simulink model "controller13_AIS"  (R2020b)
settings: Solver=FixedStepDiscrete  StartTime=0.0  StopTime=inf  RelTol=1e-3
values from neighbouring files (symbols this model uses):
  ctr = make_controller()    [setup_controller_with_functions.m]
  mdl = make_model(flight_time)    [setup_controller_with_functions.m]
  ukf_P0_flat = UKF.flatten_matrix(ukf_sys.P0)    [controller_setup_ukf.m]
  ukf_prediction_time = 0.015    [controller_setup_ukf.m]
  ukf_s0 = ukf_sys.s0    [controller_setup_ukf.m]
  ukf_sys = UKF.initialize_ukf_sys(rbt, mdl, ukf_params)    [controller_setup_ukf.m]
  ukf_use_prediction = 1    [controller_setup_ukf.m]
undefined symbols (not defined in the file or in its folder): ctr1, ctr2, DiscIntNeverNeededParam, flt, IO397, rbt1, rbt2, rsim1, rsim2, som, traj2
libraries: simulink x63, slrealtimeloglib x21, slrealtimetgmanagement x8, slrealtimeseriallib x5, speedgoatlib_fpga_analog_io x4, slrealtimeutilitieslib x3, dspfdesign x2, speedgoatlib_fpga x2, slrealtimeiplib x2, speedgoatlib_fpga_dio x1
(part 1 of 5)
settings Model: SimulationMode=external  Creator=SMRL  LastModifiedBy=SMRL
settings SolverCC: ConcurrentTasks=on  PositivePriorityOrder=on  AutoInsertRateTranBlk=on
settings DataIOCC: DSMLogging=off
settings OptimizationCC: BlockReduction=off  OptimizeBlockIOStorage=off
settings DebuggingCC: TasksWithSamePriorityMsg=none
settings HardwareCC: ProdBitPerLong=64  ProdLongLongMode=on  ProdHWDeviceType=Intel->x86-64 (Linux 64)
settings RTWCC: Description=Simulink Real-Time  SystemTargetFile=slrealtime.tlc  TemplateMakefile=slrealtime_default_tmf  Toolchain=Simulink Real-Time Toolchain  BuildConfiguration=Faster Runs  CodeExecutionProfiling=on  CodeProfilingInstrumentation=coarse  TargetLang=C++

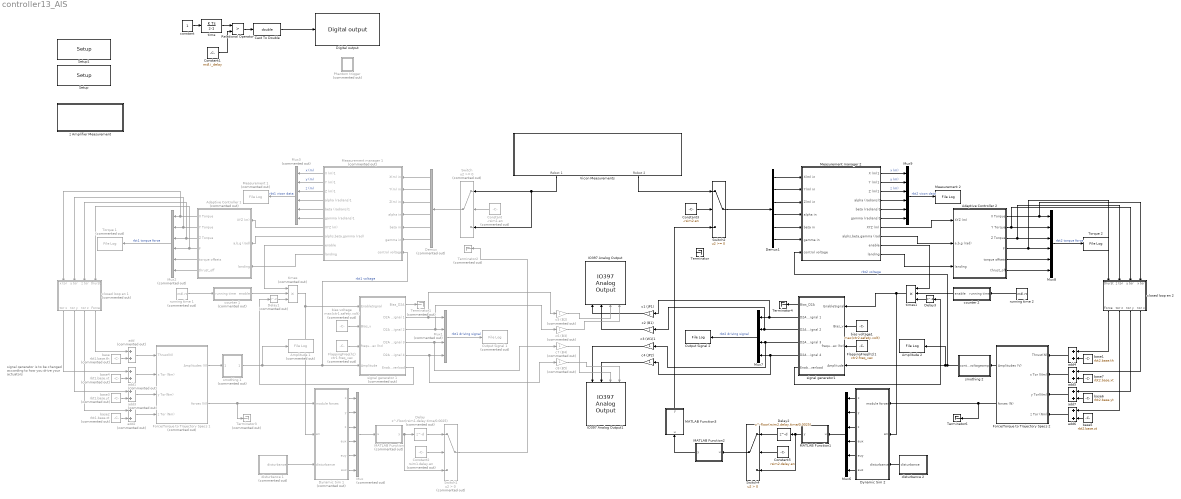
== system controller13_AIS ==
  note: signal generator is to be changed
      | according to how you drive your
      | actuators
  Adaptive Controller 1 : Subsystem  Commented=on
  Adaptive Controller 2 : Subsystem
  Amplitude 1 : slrealtimeloglib/File Log  Commented=on  decimation=1
      settings: SourceProductBaseCode=XP
  Amplitude 2 : slrealtimeloglib/File Log  decimation=1
      settings: SourceProductBaseCode=XP
  Cast To Double : DataTypeConversion  OutDataTypeStr=double
  Constant : Constant  Commented=on  Value=-rsim1.en
  Constant1 : Constant  Value=mdl.i_delay
  Constant2 : Constant  Commented=on  Value=rsim1.delay.en
  Constant3 : Constant  Value=-rsim2.en
  Constant5 : Constant  Value=rsim2.delay.en
  Delay : Delay  Commented=on  DelayLength=floor(rsim1.delay.time/0.0025)
  Delay1 : Delay  Commented=on  InitialCondition=1
  Delay2 : Delay  DelayLength=floor(rsim2.delay.time/0.0025)
  Delay3 : Delay  InitialCondition=1
  Demux : Demux  Commented=on  Outputs=6
  Demux1 : Demux  Outputs=6
  Digital output : speedgoatlib_fpga_dio/Digital output  id=2  chan=[7]  init=[0]  reset=[0]  vectorizeInput=off  ts=mdl.T  pciSlot=[11,0]  board=IO397-50k
      settings: SourceProductName=Simulink Real-Time: Speedgoat I/O Driver Library
  Dynamic Sim 1 : Subsystem  Commented=on  TreatAsAtomicUnit=on  SystemSampleTime=rsim1.mdl.T
  Dynamic Sim 2 : Subsystem  TreatAsAtomicUnit=on  SystemSampleTime=rsim2.mdl.T
  FlappingFreq(hz) : Constant  Commented=on  Value=ctr1.freq_vec  SampleTime=-1
  FlappingFreq(hz)1 : Constant  Value=ctr2.freq_vec  SampleTime=-1
  Force/Torque to Trajectory Specs 1 : Subsystem  Commented=on
  Force/Torque to Trajectory Specs 2 : Subsystem
  IO397 Analog Output : speedgoatlib_fpga_analog_io/IO397 Analog Output  id=1  chan=1:4  initVal=0  resetVal=0  ts=-1  pciSlot=[6,0]  board=IO397-50k  span=+10.8 V
      settings: SourceProductName=Simulink Real-Time: Speedgoat Library
  IO397 Analog Output1 : speedgoatlib_fpga_analog_io/IO397 Analog Output  id=2  chan=1:4  initVal=0  resetVal=0  ts=-1  pciSlot=[11,0]  board=IO397-50k  span=+10.8 V
      settings: SourceProductName=Simulink Real-Time: Speedgoat Library
  MATLAB Function : MATLAB Function  Commented=on  TreatAsAtomicUnit=on  SystemSampleTime=0.0025
  MATLAB Function1 : MATLAB Function  TreatAsAtomicUnit=on  SystemSampleTime=0.002
  MATLAB Function2 : MATLAB Function  TreatAsAtomicUnit=on  SystemSampleTime=1/500
  MATLAB Function3 : MATLAB Function  TreatAsAtomicUnit=on  SystemSampleTime=mdl.T
  Measurement 1 : slrealtimeloglib/File Log  Commented=on  decimation=1
      settings: SourceProductBaseCode=XP
  Measurement 2 : slrealtimeloglib/File Log  decimation=1
      settings: SourceProductBaseCode=XP
  Measurement manager 1 : Subsystem  Commented=on
  Measurement manager 2 : Subsystem  SystemSampleTime=mdl.T
  Mux : Mux  Commented=on  Inputs=6
  Mux1 : Mux  Commented=on
  Mux2 : Mux  Commented=on  Inputs=6
  Mux3 : Mux  Commented=on  Inputs=6
  Mux6 : Mux  Inputs=6
  Mux7 : Mux
  Mux8 : Mux  Inputs=6
  Mux9 : Mux  Inputs=6
  Output Signal 1 : slrealtimeloglib/File Log  Commented=on  decimation=1
      settings: SourceProductBaseCode=XP
  Output Signal 2 : slrealtimeloglib/File Log  decimation=1
      settings: SourceProductBaseCode=XP
  Phantom trigger : Subsystem  Commented=on
  Relational Operator : RelationalOperator  Operator=>  OutDataTypeStr=boolean  RndMeth=Simplest
  Setup : speedgoatlib_fpga/Setup/Setup  board=IO397-50k  id=2  device_id=2  frontIO=None  rearIO=None  bitstreamFile=speedgoat_IO397_50k_all_io_2.mat  rev=2.1  timestamp_string=06/12/19 11:07:30  fpgaFreq=75 MHz  fpgaTick=13.33 ns  ProgSpiFlash=off  ProgBPIFlash=off  pciSlot=[11,0]  PullRPort0=pull-up 3.3V  VioPort0=3.3V  PullRPort1=pull-up 3.3V  VioPort1=3.3V  PullRPort2=pull-up 3.3V  VioPort2=3.3V  PullRPort3=pull-up 3.3V  VioPort3=3.3V  PullRPort4=pull-up 3.3V  VioPort4=3.3V  PullRPort5=pull-up 3.3V  VioPort5=3.3V  PullRPort6=pull-up 3.3V  VioPort6=3.3V  PullRPort15=pull-up 3.3V  PullRPort31=pull-up 3.3V  PullRPort47=pull-up 3.3V  PullRPort63=pull-up 3.3V
      settings: SourceProductName=Simulink Real-Time: Speedgoat Library
  Setup1 : speedgoatlib_fpga/Setup/Setup  board=IO397-50k  id=1  device_id=1  frontIO=None  rearIO=None  bitstreamFile=speedgoat_IO397_50k_all_io_2.mat  rev=2.1  timestamp_string=06/12/19 11:07:30  fpgaFreq=75 MHz  fpgaTick=13.33 ns  ProgSpiFlash=off  ProgBPIFlash=off  pciSlot=[6,0]  PullRPort0=pull-up 3.3V  VioPort0=3.3V  PullRPort1=pull-up 3.3V  VioPort1=3.3V  PullRPort2=pull-up 3.3V  VioPort2=3.3V  PullRPort3=pull-up 3.3V  VioPort3=3.3V  PullRPort4=pull-up 3.3V  VioPort4=3.3V  PullRPort5=pull-up 3.3V  VioPort5=3.3V  PullRPort6=pull-up 3.3V  VioPort6=3.3V  PullRPort15=pull-up 3.3V  PullRPort31=pull-up 3.3V  PullRPort47=pull-up 3.3V  PullRPort63=pull-up 3.3V
      settings: SourceProductName=Simulink Real-Time: Speedgoat Library
  Switch : Switch  Commented=on
  Switch1 : Switch  Commented=on  Criteria=u2 > Threshold
  Switch2 : Switch
  Switch4 : Switch  Criteria=u2 > Threshold
  Terminator : Terminator
  Terminator1 : Terminator  Commented=on
  Terminator2 : Terminator  Commented=on
  Terminator3 : Terminator  Commented=on
  Terminator4 : Terminator
  Terminator6 : Terminator
  Torque 1 : slrealtimeloglib/File Log  Commented=on  decimation=1
      settings: SourceProductBaseCode=XP
  Torque 2 : slrealtimeloglib/File Log  decimation=1
      settings: SourceProductBaseCode=XP
  Vicon Measurements : Subsystem
  add{,1..3} (4 alike) : Sum  Commented=on
  add{4..7} (4 alike) : Sum
  base : Constant  Commented=on  Value=rbt1.base.th
  base1 : Constant  Value=rbt2.base.th
  base2 : Constant  Commented=on  Value=rbt1.base.zt
  base3 : Constant  Commented=on  Value=rbt1.base.yt
  base4 : Constant  Commented=on  Value=rbt1.base.xt
  base5 : Constant  Value=rbt2.base.zt
  base6 : Constant  Value=rbt2.base.yt
  base7 : Constant  Value=rbt2.base.xt
  bias voltage : Constant  Commented=on  Value=max(ctr1.safety.volt)
  bias voltage1 : Constant  Value=max(ctr2.safety.volt)
  c1 (JP1) : Gain
  c2 (B1) : Gain
  c3 (W1)1 : Gain
  c4 (JP2) : Gain
  c5 (B2) : Gain  Commented=on
  c6 (B3) : Gain  Commented=on
  c7 (B4) : Gain  Commented=on
  c8 (B5) : Gain  Commented=on
  closed loop en 1 : Subsystem  Commented=on
  closed loop en 2 : Subsystem
  constant : Constant
  counter 1 : Subsystem  Commented=on
  counter 2 : Subsystem
  disturbance 1 : Subsystem  Commented=on  TreatAsAtomicUnit=on  SystemSampleTime=rsim1.mdl.T
  disturbance 2 : Subsystem  TreatAsAtomicUnit=on  SystemSampleTime=rsim2.mdl.T
  running time 1 : Constant  Commented=on  Value=mdl.rt  SampleTime=-1
  running time 2 : Constant  Value=mdl.rt  SampleTime=-1
  signal generator 1 : Subsystem  Commented=on  TreatAsAtomicUnit=on  SystemSampleTime=mdl.T_high
  signal generator1 : Subsystem  TreatAsAtomicUnit=on  SystemSampleTime=mdl.T_high
  smothing 1 : Subsystem  Commented=on
  smothing 2 : Subsystem
  time : DiscreteIntegrator  gainval=1  SampleTime=-1  UpperSaturationLimit=1  LowerSaturationLimit=0  ICPrevOutput=DiscIntNeverNeededParam  ICPrevScaledInput=DiscIntNeverNeededParam
  times : Product  Commented=on  Inputs=3  RndMeth=Zero
  times1 : Product  Inputs=3  RndMeth=Zero
  z Amplifier Measurement : Subsystem
  wires:
  add3/1 -> Force/Torque to Trajectory Specs 1/3(y Tor(Nm))
  Force/Torque to Trajectory Specs 1/2(forces (N)) -> Dynamic Sim 1/1(module forces), Terminator3/1
  Adaptive Controller 1/3(Z Torque) -> Mux2/3, closed loop en 1/3(z tor)
  Mux3/1 -> Measurement 1/1  "rbt1 vicon data"
  Adaptive Controller 1/2(Y Torque) -> Mux2/2, closed loop en 1/2(y tor)
  Adaptive Controller 1/1(X Torque) -> Mux2/1, closed loop en 1/1(x tor)
  signal generator 1/5(D2A DriveSignal 4) -> c8 (B5)/1, Mux1/4
  Adaptive Controller 1/5(" torque offsets") -> Mux2/5
  Measurement manager 1/5(beta (radians)1) -> Mux3/5
  signal generator 1/4(D2A DriveSignal 3) -> c7 (B4)/1, Mux1/3
  Adaptive Controller 1/4(" F") -> Mux2/4, closed loop en 1/4(thurst)
  Measurement manager 1/6(gamma (radians)1) -> Mux3/6
  add2/1 -> Force/Torque to Trajectory Specs 1/4(z Tor (Nm))
  Measurement manager 1/4(alpha (radians)1) -> Mux3/4
  Adaptive Controller 1/6(thrust_off) -> Mux2/6
  closed loop en 1/1(tor x) -> add1/1
  base3/1 -> add3/2
  base2/1 -> add2/2
  Mux1/1 -> Output Signal 1/1  "rbt1 driving signal"
  closed loop en 1/4(Force) -> add/1
  base/1 -> add/2
  Measurement manager 1/8(alphs,beta,gamma (rad)) -> Adaptive Controller 1/2(a,b,g (rad))
  signal generator 1/2(D2A DriveSignal 1) -> Mux1/1, c5 (B2)/1
  closed loop en 1/2(tor y) -> add3/1
  signal generator 1/3(D2A DriveSignal 2) -> c6 (B3)/1, Mux1/2
  Force/Torque to Trajectory Specs 1/1(Amplitudes (V)) -> smothing 1/1(amp)
  FlappingFreq(hz)/1 -> signal generator 1/3(frequency_vec (hz))
  Measurement manager 1/1(X (m)1) -> Mux3/1  "x (m)"
  Measurement manager 1/7(XYZ (m)) -> Adaptive Controller 1/1(XYZ (m))
  Measurement manager 1/3(Z (m)1) -> Mux3/3  "z (m)"
  base4/1 -> add1/2
  closed loop en 1/3(tor z) -> add2/1
  add1/1 -> Force/Torque to Trajectory Specs 1/2(x Tor (Nm))
  bias voltage/1 -> signal generator 1/2(Bias_v)
  counter 1/1(enable) -> times/2
  add/1 -> Force/Torque to Trajectory Specs 1/1(Thrust(N))
  Measurement manager 1/2(Y (m)1) -> Mux3/2  "y (m)"
  running time 1/1 -> counter 1/1(running time)
  Mux2/1 -> Torque 1/1  "rbt1 torque force"
  signal generator 1/1(Bias_D2A) -> Terminator1/1
  Dynamic Sim 1/3(z) -> Mux/3
  Dynamic Sim 1/2(y) -> Mux/2
  Dynamic Sim 1/1(x) -> Mux/1
  Dynamic Sim 1/4(eux) -> Mux/4
  Dynamic Sim 1/5(euy) -> Mux/5
  Dynamic Sim 1/6(euz) -> Mux/6
  Demux/1 -> Measurement manager 1/1(X(m) in)
  Demux/2 -> Measurement manager 1/2(Y(m) in)
  Demux/3 -> Measurement manager 1/3(Z(m) in)
  Demux/4 -> Measurement manager 1/4(alpha in)
  Demux/5 -> Measurement manager 1/5(beta in)
  Demux/6 -> Measurement manager 1/6(gamma in)
  Constant/1 -> Switch/2
  disturbance 1/1(disturbance) -> Dynamic Sim 1/3(disturbance)
  times/1 -> signal generator 1/1(EnableSignal), Dynamic Sim 1/2(en)
  Switch/1 -> Demux/1
  Switch1/1 -> Terminator2/1
  Cast To Double/1 -> Digital output/1
  constant/1 -> time/1
  time/1 -> Relational Operator/1
  Relational Operator/1 -> Cast To Double/1
  Constant1/1 -> Relational Operator/2
  Measurement manager 1/10(landing) -> Adaptive Controller 1/3(landing)
  signal generator 1/6(Enable overload) -> Delay1/1
  Delay1/1 -> times/3
  smothing 1/1(control voltage) -> signal generator 1/4(Amplitude), Measurement manager 1/7(control voltage), Amplitude 1/1  "rbt1 voltage"
  Measurement manager 1/9(enable) -> times/1
  Mux/1 -> MATLAB Function/1(u)
  Delay/1 -> Switch1/1
  Constant2/1 -> Switch1/2
  MATLAB Function/1(y) -> Switch1/3, Delay/1
  Constant3/1 -> Switch2/2
  MATLAB Function1/1(y) -> Switch4/3, Delay2/1
  Mux6/1 -> MATLAB Function1/1(u)
  smothing 2/1(control voltage) -> signal generator1/4(Amplitude), Amplitude 2/1, Measurement manager 2/7(control voltage)  "rbt2 voltage"
  Measurement manager 2/10(landing) -> Adaptive Controller 2/3(landing)
  Demux1/2 -> Measurement manager 2/2(Y(m) in)
  Measurement manager 2/4(alpha (radians)1) -> Mux9/4
  closed loop en 2/2(tor y) -> add7/1
  Demux1/1 -> Measurement manager 2/1(X(m) in)
  Demux1/5 -> Measurement manager 2/5(beta in)
  Delay3/1 -> times1/3
  Delay2/1 -> Switch4/1
  Measurement manager 2/9(enable) -> times1/1
  Constant5/1 -> Switch4/2
  disturbance 2/1(disturbance) -> Dynamic Sim 2/3(disturbance)
  times1/1 -> signal generator1/1(EnableSignal), Dynamic Sim 2/2(en)
  signal generator1/6(Enable overload) -> Delay3/1
  Mux8/1 -> Torque 2/1  "rbt2 torque force"
  signal generator1/3(D2A DriveSignal 2) -> c2 (B1)/1, Mux7/2
  closed loop en 2/3(tor z) -> add6/1
  Demux1/6 -> Measurement manager 2/6(gamma in)
  Dynamic Sim 2/5(euy) -> Mux6/5
  Measurement manager 2/1(X (m)1) -> Mux9/1  "x (m)"
  add6/1 -> Force/Torque to Trajectory Specs 2/4(z Tor (Nm))
  closed loop en 2/1(tor x) -> add5/1
  Dynamic Sim 2/4(eux) -> Mux6/4
  Adaptive Controller 2/6(thrust_off) -> Mux8/6
  Dynamic Sim 2/2(y) -> Mux6/2
  Dynamic Sim 2/1(x) -> Mux6/1
  counter 2/1(enable) -> times1/2
  signal generator1/4(D2A DriveSignal 3) -> c3 (W1)1/1, Mux7/3
  running time 2/1 -> counter 2/1(running time)
  signal generator1/1(Bias_D2A) -> Terminator4/1
  Measurement manager 2/2(Y (m)1) -> Mux9/2  "y (m)"
  Measurement manager 2/5(beta (radians)1) -> Mux9/5
  closed loop en 2/4(Force) -> add4/1
  add4/1 -> Force/Torque to Trajectory Specs 2/1(Thrust(N))
  bias voltage1/1 -> signal generator1/2(Bias_v)
  Adaptive Controller 2/5(" torque offsets") -> Mux8/5
  Dynamic Sim 2/6(euz) -> Mux6/6
  base6/1 -> add7/2
  base5/1 -> add6/2
  Measurement manager 2/6(gamma (radians)1) -> Mux9/6
  base7/1 -> add5/2
  Measurement manager 2/3(Z (m)1) -> Mux9/3  "z (m)"
  Adaptive Controller 2/4(" F") -> Mux8/4, closed loop en 2/4(thurst)
  Measurement manager 2/7(XYZ (m)) -> Adaptive Controller 2/1(XYZ (m))
  Force/Torque to Trajectory Specs 2/2(forces (N)) -> Dynamic Sim 2/1(module forces), Terminator6/1
  Adaptive Controller 2/1(X Torque) -> closed loop en 2/1(x tor), Mux8/1
  add5/1 -> Force/Torque to Trajectory Specs 2/2(x Tor (Nm))
  add7/1 -> Force/Torque to Trajectory Specs 2/3(y Tor(Nm))
  base1/1 -> add4/2
  Mux7/1 -> Output Signal 2/1  "rbt2 driving signal"
  Dynamic Sim 2/3(z) -> Mux6/3
  Mux9/1 -> Measurement 2/1  "rbt2 vicon data"
  Force/Torque to Trajectory Specs 2/1(Amplitudes (V)) -> smothing 2/1(amp)
  Demux1/3 -> Measurement manager 2/3(Z(m) in)
  Measurement manager 2/8(alphs,beta,gamma (rad)) -> Adaptive Controller 2/2(a,b,g (rad))
  Adaptive Controller 2/2(Y Torque) -> closed loop en 2/2(y tor), Mux8/2
  signal generator1/5(D2A DriveSignal 4) -> Mux7/4, c4 (JP2)/1
  Adaptive Controller 2/3(Z Torque) -> closed loop en 2/3(z tor), Mux8/3
  FlappingFreq(hz)1/1 -> signal generator1/3(frequency_vec (hz))
  Demux1/4 -> Measurement manager 2/4(alpha in)
  Switch2/1 -> Demux1/1
  Switch4/1 -> MATLAB Function2/1(u)
  Vicon Measurements/2(Robot 2) -> Switch2/1
  Vicon Measurements/1(Robot 1) -> Switch/3, Switch/1
  signal generator1/2(D2A DriveSignal 1) -> c1 (JP1)/1, Mux7/1
  c1 (JP1)/1 -> IO397 Analog Output/1
  c2 (B1)/1 -> IO397 Analog Output/2
  c3 (W1)1/1 -> IO397 Analog Output1/1
  c4 (JP2)/1 -> IO397 Analog Output1/2
  c5 (B2)/1 -> IO397 Analog Output/3
  c6 (B3)/1 -> IO397 Analog Output/4
  c7 (B4)/1 -> IO397 Analog Output1/3
  c8 (B5)/1 -> IO397 Analog Output1/4
  MATLAB Function2/1(y) -> MATLAB Function3/1(u)
  MATLAB Function3/1(y) -> Switch2/3

== system controller13_AIS/Adaptive Controller 1 ==
  XYZ (m) : Inport
  a,b,g (rad) : Inport  Port=2
  landing : Inport  Port=3
  Mux : Mux
  Overload Options : slrealtimetgmanagement/Overload Options  startupDur=10  startupDurSrc=Tunable Parameter  maxOverload=10  maxOverloadSrc=Tunable Parameter  TETFlag=on
      settings: SourceProductBaseCode=XP
  Terminator : Terminator
  Terminator1 : Terminator
  Terminator2 : Terminator
  adaptive setpoint rd : MATLAB Function  TreatAsAtomicUnit=on  SystemSampleTime=mdl.T
  adaptive system : Subsystem
  attitude and thrust controller : Subsystem
  observer : Subsystem
  observer_log : slrealtimeloglib/File Log  decimation=1
      settings: SourceProductBaseCode=XP
  observer_mux : Mux  Inputs=5
  rd : slrealtimeloglib/File Log  decimation=1
      settings: SourceProductBaseCode=XP
  rd_mux : Mux  Inputs=2
  saturation : MATLAB Function  TreatAsAtomicUnit=on
  somersault_phase : MATLAB Function  TreatAsAtomicUnit=on
  time : Subsystem
  X Torque : Outport
  Y Torque : Outport  Port=2
  Z Torque : Outport  Port=3
  " F" : Outport  Port=4
  " torque offsets" : Outport  Port=5
  thrust_off : Outport  Port=6
  wires:
  XYZ (m)/1 -> observer/1(xyz)
  observer/1(r) -> adaptive setpoint rd/2(r), attitude and thrust controller/1(r)
  observer/2(r_dot) -> observer_mux/1, adaptive setpoint rd/3(r_d), attitude and thrust controller/2(r_dot)
  observer/3(r_dotdot) -> observer_mux/2, attitude and thrust controller/3(r_dotdot)
  a,b,g (rad)/1 -> attitude and thrust controller/12(euler angle), observer/2(euler)
  observer/4(R) -> observer_mux/3, attitude and thrust controller/4(R)
  saturation/1(X_roll) -> Mux/1, X Torque/1
  saturation/2(Y_pitch) -> Mux/2, Y Torque/1
  saturation/3(Z_yaw) -> Mux/3, Z Torque/1
  saturation/4(Force) -> " F"/1, Mux/4
  attitude and thrust controller/4(F) -> saturation/4(Th)
  attitude and thrust controller/5(att_e) -> adaptive system/1(att_e)
  adaptive system/1(" tor_off") -> " torque offsets"/1
  adaptive system/2(th_off) -> thrust_off/1
  adaptive system/3(int_e) -> attitude and thrust controller/11(int_e)
  adaptive setpoint rd/1(rd) -> rd_mux/1, attitude and thrust controller/6(rd)  "rd"
  adaptive setpoint rd/2(rd_d) -> rd_mux/2, attitude and thrust controller/7(rd_d)
  adaptive setpoint rd/3(rd_dd) -> attitude and thrust controller/8(rd_dd)
  adaptive setpoint rd/4(rd_ddd) -> attitude and thrust controller/9(rd_ddd)
  adaptive setpoint rd/5(rd_dddd) -> attitude and thrust controller/10(rd_dddd)
  time/1(real times) -> somersault_phase/1(time), adaptive setpoint rd/1(time)
  attitude and thrust controller/3(torque_z) -> saturation/3(z_yaw)
  attitude and thrust controller/2(torque_y) -> saturation/2(y_pitch)
  attitude and thrust controller/1(torque_x) -> saturation/1(x_roll)
  observer/6(Rdot) -> observer_mux/5, Terminator/1
  observer/5(Omega) -> observer_mux/4, attitude and thrust controller/5(Omega)
  attitude and thrust controller/6(alt_e) -> adaptive system/2(alt_e)
  somersault_phase/1(som_phase) -> adaptive setpoint rd/5(som_ph), saturation/5(som_phase)
  landing/1 -> adaptive setpoint rd/4(landing)
  observer_mux/1 -> observer_log/1  "rbt1 observer"
  rd_mux/1 -> rd/1  "rbt1 trajectory"
  Mux/1 -> Overload Options/1
  Overload Options/2 -> Terminator1/1  "T/F TET"
  Overload Options/1 -> Terminator2/1  "T/F count"

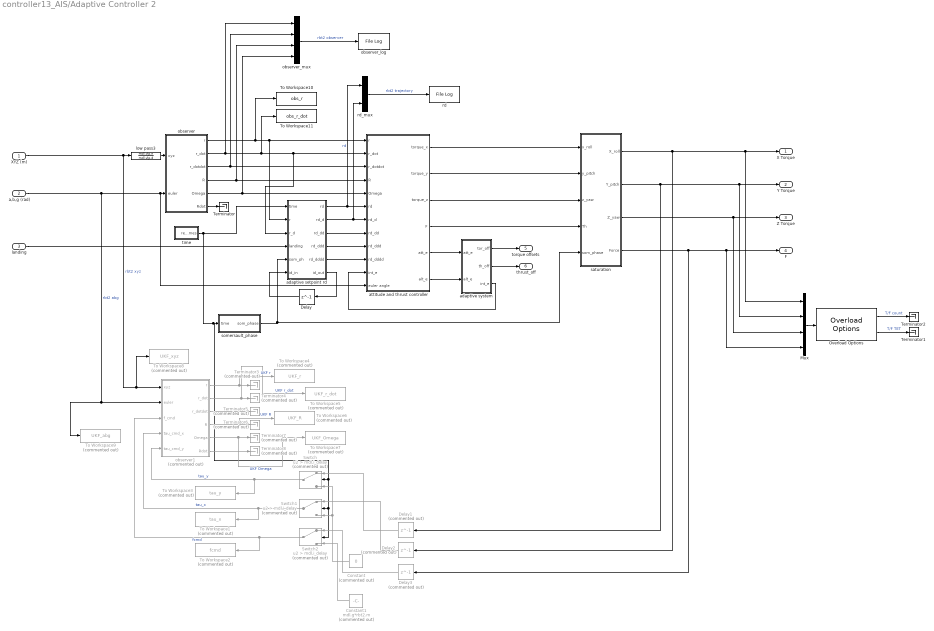
== system controller13_AIS/Adaptive Controller 2 ==
  XYZ (m) : Inport
  a,b,g (rad) : Inport  Port=2
  landing : Inport  Port=3
  Constant : Constant  Commented=on  Value=0
  Constant1 : Constant  Commented=on  Value=mdl.g*rbt2.m
  Delay : Delay  DelayLength=1  InitialCondition=1
  Delay1 : Delay  Commented=on  DelayLength=1  InitialCondition=0
  Delay2 : Delay  Commented=on  DelayLength=1  InitialCondition=0
  Delay3 : Delay  Commented=on  DelayLength=1  InitialCondition=0
  Mux : Mux
  Overload Options : slrealtimetgmanagement/Overload Options  startupDur=100  startupDurSrc=Tunable Parameter  maxOverload=10  maxOverloadSrc=Tunable Parameter  TETFlag=on
      settings: SourceProductBaseCode=XP
  Switch : Switch  Commented=on  Criteria=u2 > Threshold  Threshold=mdl.i_delay
  Switch1 : Switch  Commented=on  Criteria=u2 > Threshold  Threshold=mdl.i_delay
  Switch2 : Switch  Commented=on  Criteria=u2 > Threshold  Threshold=mdl.i_delay
  Terminator : Terminator
  Terminator1 : Terminator
  Terminator2 : Terminator
  Terminator{3..8} (6 alike) : Terminator  Commented=on
  To Workspace1 : ToWorkspace  Commented=on  VariableName=tau_x  SaveFormat=Timeseries  SampleTime=-1
  To Workspace10 : ToWorkspace  VariableName=obs_r  SaveFormat=Timeseries  SampleTime=-1
  To Workspace11 : ToWorkspace  VariableName=obs_r_dot  SaveFormat=Timeseries  SampleTime=-1
  To Workspace2 : ToWorkspace  Commented=on  VariableName=fcmd  SaveFormat=Timeseries  SampleTime=-1
  To Workspace3 : ToWorkspace  Commented=on  VariableName=tau_y  SaveFormat=Timeseries  SampleTime=-1
  To Workspace4 : ToWorkspace  Commented=on  VariableName=UKF_r  SaveFormat=Timeseries  SampleTime=-1
  To Workspace5 : ToWorkspace  Commented=on  VariableName=UKF_r_dot  SaveFormat=Timeseries  SampleTime=-1
  To Workspace6 : ToWorkspace  Commented=on  VariableName=UKF_R  SaveFormat=Timeseries  SampleTime=-1
  To Workspace7 : ToWorkspace  Commented=on  VariableName=UKF_Omega  SaveFormat=Timeseries  SampleTime=-1
  To Workspace8 : ToWorkspace  Commented=on  VariableName=UKF_xyz  SaveFormat=Timeseries  SampleTime=-1
  To Workspace9 : ToWorkspace  Commented=on  VariableName=UKF_abg  SaveFormat=Timeseries  SampleTime=-1
  adaptive setpoint rd : MATLAB Function  TreatAsAtomicUnit=on  SystemSampleTime=mdl.T
  adaptive system : Subsystem
  attitude and thrust controller : Subsystem
  low pass3 : DiscreteTransferFcn  Numerator=mdl.vlp.n  Denominator=mdl.vlp.d
  observer : Subsystem
  observer1 : Subsystem  Commented=on
  observer_log : slrealtimeloglib/File Log  decimation=1
      settings: SourceProductBaseCode=XP
  observer_mux : Mux
  rd : slrealtimeloglib/File Log  decimation=1
      settings: SourceProductBaseCode=XP
  rd_mux : Mux  Inputs=2
  saturation : MATLAB Function  TreatAsAtomicUnit=on
  somersault_phase : MATLAB Function  TreatAsAtomicUnit=on
  time : Subsystem
  X Torque : Outport
  Y Torque : Outport  Port=2
  Z Torque : Outport  Port=3
  " F" : Outport  Port=4
  " torque offsets" : Outport  Port=5
  thrust_off : Outport  Port=6
  wires:
  XYZ (m)/1 -> To Workspace8/1, observer1/1(xyz), low pass3/1  "rbt2 xyz"
  observer/1(r) -> To Workspace10/1, attitude and thrust controller/1(r), adaptive setpoint rd/2(r)
  observer/2(r_dot) -> observer_mux/1, To Workspace11/1, adaptive setpoint rd/3(r_d), attitude and thrust controller/2(r_dot)
  observer/3(r_dotdot) -> observer_mux/2, attitude and thrust controller/3(r_dotdot)
  a,b,g (rad)/1 -> observer1/2(euler), To Workspace9/1, attitude and thrust controller/12(euler angle), observer/2(euler)  "rbt2 abg"
  observer/4(R) -> observer_mux/3, attitude and thrust controller/4(R)
  saturation/1(X_roll) -> Mux/1, X Torque/1, Delay2/1
  saturation/2(Y_pitch) -> Delay1/1, Mux/2, Y Torque/1
  saturation/3(Z_yaw) -> Mux/3, Z Torque/1
  saturation/4(Force) -> " F"/1, Mux/4, Delay3/1
  attitude and thrust controller/4(F) -> saturation/4(Th)
  attitude and thrust controller/5(att_e) -> adaptive system/1(att_e)
  adaptive system/1(" tor_off") -> " torque offsets"/1
  adaptive system/2(th_off) -> thrust_off/1
  adaptive system/3(int_e) -> attitude and thrust controller/11(int_e)
  adaptive setpoint rd/1(rd) -> rd_mux/1, attitude and thrust controller/6(rd)  "rd"
  adaptive setpoint rd/2(rd_d) -> rd_mux/2, attitude and thrust controller/7(rd_d)
  adaptive setpoint rd/3(rd_dd) -> attitude and thrust controller/8(rd_dd)
  adaptive setpoint rd/4(rd_ddd) -> attitude and thrust controller/9(rd_ddd)
  adaptive setpoint rd/5(rd_dddd) -> attitude and thrust controller/10(rd_dddd)
  time/1(real times) -> Switch/2, Switch2/2, Switch1/2, somersault_phase/1(time), adaptive setpoint rd/1(time)
  attitude and thrust controller/3(torque_z) -> saturation/3(z_yaw)
  attitude and thrust controller/2(torque_y) -> saturation/2(y_pitch)
  attitude and thrust controller/1(torque_x) -> saturation/1(x_roll)
  observer/6(Rdot) -> Terminator/1
  observer/5(Omega) -> observer_mux/4, attitude and thrust controller/5(Omega)
  attitude and thrust controller/6(alt_e) -> adaptive system/2(alt_e)
  somersault_phase/1(som_phase) -> saturation/5(som_phase), adaptive setpoint rd/5(som_ph)
  landing/1 -> adaptive setpoint rd/4(landing)
  observer_mux/1 -> observer_log/1  "rbt2 observer"
  rd_mux/1 -> rd/1  "rbt2 trajectory"
  Mux/1 -> Overload Options/1
  Overload Options/2 -> Terminator1/1  "T/F TET"
  Overload Options/1 -> Terminator2/1  "T/F count"
  adaptive setpoint rd/6(id_out) -> Delay/1
  Delay/1 -> adaptive setpoint rd/6(id_in)
  observer1/1(r) -> To Workspace4/1, Terminator3/1  "UKF r"
  observer1/2(r_dot) -> To Workspace5/1, Terminator4/1  "UKF r_dot"
  observer1/3(r_dotdot) -> Terminator5/1
  observer1/4(R) -> To Workspace6/1, Terminator6/1  "UKF R"
  observer1/5(Omega) -> To Workspace7/1, Terminator7/1  "UKF Omega"
  observer1/6(Rdot) -> Terminator8/1
  low pass3/1 -> observer/1(xyz)
  Switch/1 -> To Workspace3/1, observer1/5(tau_cmd_y)  "tau_y"
  Delay1/1 -> Switch/1
  Switch1/1 -> To Workspace1/1, observer1/4(tau_cmd_x)  "tau_x"
  Delay2/1 -> Switch1/1
  Switch2/1 -> To Workspace2/1, observer1/3(f_cmd)  "fcmd"
  Delay3/1 -> Switch2/1
  Constant/1 -> Switch/3, Switch1/3
  Constant1/1 -> Switch2/3

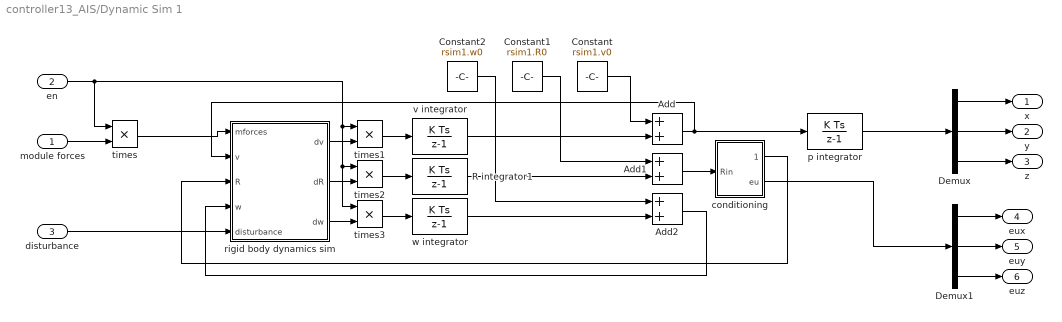
== system controller13_AIS/Dynamic Sim 1 ==
  module forces : Inport
  en : Inport  Port=2
  disturbance : Inport  Port=3
  Add : Sum
  Add1 : Sum
  Add2 : Sum
  Constant : Constant  Value=rsim1.v0
  Constant1 : Constant  Value=rsim1.R0
  Constant2 : Constant  Value=rsim1.w0
  Demux : Demux  Outputs=3
  Demux1 : Demux  Outputs=3
  R integrator1 : DiscreteIntegrator  gainval=1  SampleTime=-1  UpperSaturationLimit=1  LowerSaturationLimit=0  ICPrevOutput=DiscIntNeverNeededParam  ICPrevScaledInput=DiscIntNeverNeededParam
  conditioning : MATLAB Function  TreatAsAtomicUnit=on
  p integrator : DiscreteIntegrator  gainval=1  InitialCondition=rsim1.p0  SampleTime=-1  UpperSaturationLimit=1  LowerSaturationLimit=0  ICPrevOutput=DiscIntNeverNeededParam  ICPrevScaledInput=DiscIntNeverNeededParam
  rigid body dynamics sim : MATLAB Function  TreatAsAtomicUnit=on
  times{,1..3} (4 alike) : Product  RndMeth=Zero
  v integrator : DiscreteIntegrator  gainval=1  SampleTime=-1  UpperSaturationLimit=1  LowerSaturationLimit=0  ICPrevOutput=DiscIntNeverNeededParam  ICPrevScaledInput=DiscIntNeverNeededParam
  w integrator : DiscreteIntegrator  gainval=1  SampleTime=-1  UpperSaturationLimit=1  LowerSaturationLimit=0  ICPrevOutput=DiscIntNeverNeededParam  ICPrevScaledInput=DiscIntNeverNeededParam
  x : Outport  VectorParamsAs1DForOutWhenUnconnected=off
  y : Outport  Port=2  VectorParamsAs1DForOutWhenUnconnected=off
  z : Outport  Port=3  VectorParamsAs1DForOutWhenUnconnected=off
  eux : Outport  Port=4  VectorParamsAs1DForOutWhenUnconnected=off
  euy : Outport  Port=5  VectorParamsAs1DForOutWhenUnconnected=off
  euz : Outport  Port=6  VectorParamsAs1DForOutWhenUnconnected=off
  wires:
  Demux1/1 -> eux/1
  Demux1/2 -> euy/1
  Demux/3 -> z/1
  conditioning/2(eu) -> Demux1/1
  conditioning/1(Rout) -> rigid body dynamics sim/3(R)
  p integrator/1 -> Demux/1
  Demux1/3 -> euz/1
  Demux/1 -> x/1
  Demux/2 -> y/1
  v integrator/1 -> Add/2
  Constant/1 -> Add/1
  Constant1/1 -> Add1/1
  R integrator1/1 -> Add1/2
  Constant2/1 -> Add2/1
  w integrator/1 -> Add2/2
  Add1/1 -> conditioning/1(Rin)
  Add2/1 -> rigid body dynamics sim/4(w)
  Add/1 -> rigid body dynamics sim/2(v), p integrator/1
  en/1 -> times2/1, times3/1, times1/1, times/1
  module forces/1 -> times/2
  times/1 -> rigid body dynamics sim/1(mforces)
  times1/1 -> v integrator/1
  rigid body dynamics sim/1(dv) -> times1/2
  rigid body dynamics sim/2(dR) -> times2/2
  rigid body dynamics sim/3(dw) -> times3/2
  times2/1 -> R integrator1/1
  times3/1 -> w integrator/1
  disturbance/1 -> rigid body dynamics sim/5(disturbance)

== system controller13_AIS/Dynamic Sim 2 ==
  module forces : Inport
  en : Inport  Port=2
  disturbance : Inport  Port=3
  Add : Sum
  Add1 : Sum
  Add2 : Sum
  Constant : Constant  Value=rsim2.v0
  Constant1 : Constant  Value=rsim2.R0
  Constant2 : Constant  Value=rsim2.w0
  Demux : Demux  Outputs=3
  Demux1 : Demux  Outputs=3
  R integrator1 : DiscreteIntegrator  gainval=1  SampleTime=-1  UpperSaturationLimit=1  LowerSaturationLimit=0  ICPrevOutput=DiscIntNeverNeededParam  ICPrevScaledInput=DiscIntNeverNeededParam
  conditioning : MATLAB Function  TreatAsAtomicUnit=on
  p integrator : DiscreteIntegrator  gainval=1  InitialCondition=rsim2.p0  SampleTime=-1  UpperSaturationLimit=1  LowerSaturationLimit=0  ICPrevOutput=DiscIntNeverNeededParam  ICPrevScaledInput=DiscIntNeverNeededParam
  rigid body dynamics sim : MATLAB Function  TreatAsAtomicUnit=on
  times{,1..3} (4 alike) : Product  RndMeth=Zero
  v integrator : DiscreteIntegrator  gainval=1  SampleTime=-1  UpperSaturationLimit=1  LowerSaturationLimit=0  ICPrevOutput=DiscIntNeverNeededParam  ICPrevScaledInput=DiscIntNeverNeededParam
  w integrator : DiscreteIntegrator  gainval=1  SampleTime=-1  UpperSaturationLimit=1  LowerSaturationLimit=0  ICPrevOutput=DiscIntNeverNeededParam  ICPrevScaledInput=DiscIntNeverNeededParam
  x : Outport  VectorParamsAs1DForOutWhenUnconnected=off
  y : Outport  Port=2  VectorParamsAs1DForOutWhenUnconnected=off
  z : Outport  Port=3  VectorParamsAs1DForOutWhenUnconnected=off
  eux : Outport  Port=4  VectorParamsAs1DForOutWhenUnconnected=off
  euy : Outport  Port=5  VectorParamsAs1DForOutWhenUnconnected=off
  euz : Outport  Port=6  VectorParamsAs1DForOutWhenUnconnected=off
  wires:
  Demux1/1 -> eux/1
  Demux1/2 -> euy/1
  Demux/3 -> z/1
  conditioning/2(eu) -> Demux1/1
  conditioning/1(Rout) -> rigid body dynamics sim/3(R)
  p integrator/1 -> Demux/1
  Demux1/3 -> euz/1
  Demux/1 -> x/1
  Demux/2 -> y/1
  v integrator/1 -> Add/2
  Constant/1 -> Add/1
  Constant1/1 -> Add1/1
  R integrator1/1 -> Add1/2
  Constant2/1 -> Add2/1
  w integrator/1 -> Add2/2
  Add1/1 -> conditioning/1(Rin)
  Add2/1 -> rigid body dynamics sim/4(w)
  Add/1 -> rigid body dynamics sim/2(v), p integrator/1
  en/1 -> times2/1, times3/1, times1/1, times/1
  module forces/1 -> times/2
  times/1 -> rigid body dynamics sim/1(mforces)
  times1/1 -> v integrator/1
  rigid body dynamics sim/1(dv) -> times1/2
  rigid body dynamics sim/2(dR) -> times2/2
  rigid body dynamics sim/3(dw) -> times3/2
  times2/1 -> R integrator1/1
  times3/1 -> w integrator/1
  disturbance/1 -> rigid body dynamics sim/5(disturbance)

== system controller13_AIS/Force//Torque to Trajectory Specs 1 ==
  Thrust(N) : Inport
  x Tor (Nm) : Inport  Port=2
  y Tor(Nm) : Inport  Port=3
  z Tor (Nm) : Inport  Port=4
  force/torque to module thrust : Subsystem
  nominal desired voltage : Subsystem
  Amplitudes (V) : Outport
  forces (N) : Outport  Port=2
  wires:
  Thrust(N)/1 -> force/torque to module thrust/1(thrust)
  y Tor(Nm)/1 -> force/torque to module thrust/3(y Tq)
  z Tor (Nm)/1 -> force/torque to module thrust/4(z Tq)
  force/torque to module thrust/1(module thrusts (1-4)) -> forces (N)/1, nominal desired voltage/1(Force)
  x Tor (Nm)/1 -> force/torque to module thrust/2(x Tq)
  nominal desired voltage/1(Voltages) -> Amplitudes (V)/1

== system controller13_AIS/Force//Torque to Trajectory Specs 2 ==
  Thrust(N) : Inport
  x Tor (Nm) : Inport  Port=2
  y Tor(Nm) : Inport  Port=3
  z Tor (Nm) : Inport  Port=4
  Overload Options : slrealtimetgmanagement/Overload Options  startupDur=1000  startupDurSrc=Tunable Parameter  maxOverload=1000  maxOverloadSrc=Tunable Parameter  TETFlag=on
      settings: SourceProductBaseCode=XP
  Terminator1 : Terminator
  Terminator2 : Terminator
  force/torque to module thrust : Subsystem
  nominal desired voltage : Subsystem
  Amplitudes (V) : Outport
  forces (N) : Outport  Port=2
  wires:
  Thrust(N)/1 -> force/torque to module thrust/1(thrust)
  y Tor(Nm)/1 -> force/torque to module thrust/3(y Tq)
  z Tor (Nm)/1 -> force/torque to module thrust/4(z Tq)
  force/torque to module thrust/1(module thrusts (1-4)) -> forces (N)/1, nominal desired voltage/1(Force)
  x Tor (Nm)/1 -> force/torque to module thrust/2(x Tq)
  nominal desired voltage/1(Voltages) -> Overload Options/1, Amplitudes (V)/1
  Overload Options/1 -> Terminator2/1  "F2V count"
  Overload Options/2 -> Terminator1/1  "F2V TET"

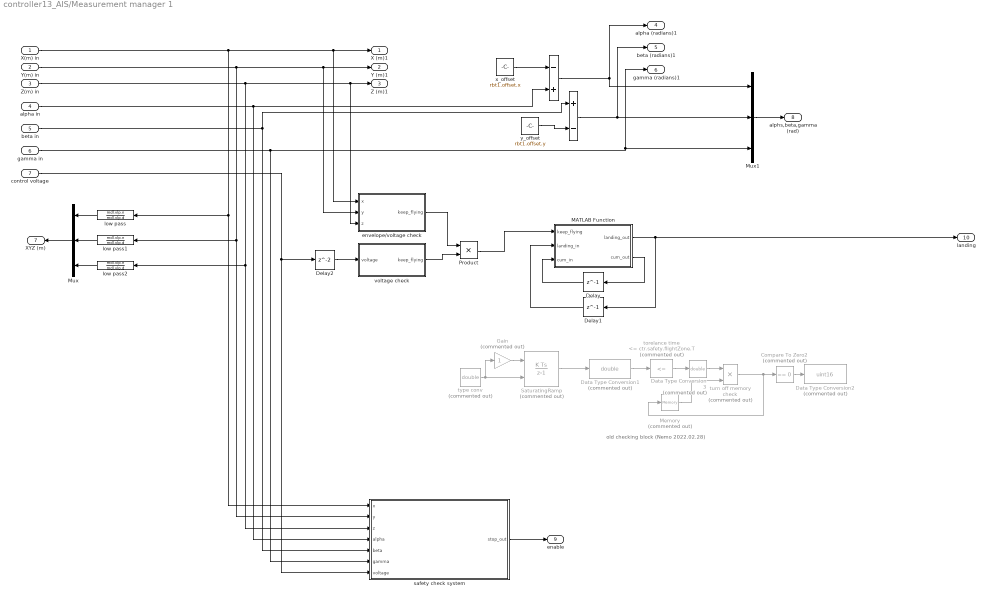
== system controller13_AIS/Measurement manager 1 ==
  note: old checking block (Nemo 2022.02.28)
  X(m) in : Inport
  Y(m) in : Inport  Port=2
  Z(m) in : Inport  Port=3
  alpha in : Inport  Port=4
  beta in : Inport  Port=5
  gamma in : Inport  Port=6
  control voltage : Inport  Port=7
  " " : Sum  Inputs=-+
  "  " : Sum  Inputs=+-
  Compare To Zero2 : simulink/Logic and Bit Operations/Compare To Zero  Commented=on  relop===  OutDataTypeStr=uint8
  Data Type Conversion1 : DataTypeConversion  Commented=on  OutDataTypeStr=double
  Data Type Conversion2 : DataTypeConversion  Commented=on  OutDataTypeStr=uint16
  Data Type Conversion3 : DataTypeConversion  Commented=on  OutDataTypeStr=double
  Delay : Delay  DelayLength=1
  Delay1 : Delay  DelayLength=1
  Delay2 : Delay  SampleTime=mdl.T
  Gain : Gain  Commented=on
  MATLAB Function : MATLAB Function  TreatAsAtomicUnit=on
  Memory : Memory  Commented=on  InitialCondition=1
  Mux : Mux  Inputs=3
  Mux1 : Mux  Inputs=3
  Product : Product
  SaturatingRamp : DiscreteIntegrator  Commented=on  gainval=1  ExternalReset=falling  SampleTime=-1  UpperSaturationLimit=1  LowerSaturationLimit=0  ICPrevOutput=DiscIntNeverNeededParam  ICPrevScaledInput=DiscIntNeverNeededParam
  envelope/voltage check : MATLAB Function  TreatAsAtomicUnit=on
  low pass : DiscreteTransferFcn  Numerator=mdl.vlp.n  Denominator=mdl.vlp.d
  low pass1 : DiscreteTransferFcn  Numerator=mdl.vlp.n  Denominator=mdl.vlp.d
  low pass2 : DiscreteTransferFcn  Numerator=mdl.vlp.n  Denominator=mdl.vlp.d
  safety check system : Subsystem
  torelance time : simulink/Logic and Bit Operations/Compare To Constant  Commented=on  relop=<=  const=ctr.safety.flightZone.T  OutDataTypeStr=uint8
  turn off memory check : Product  Commented=on  RndMeth=Zero
  type conv : DataTypeConversion  Commented=on  OutDataTypeStr=double
  voltage check : MATLAB Function  TreatAsAtomicUnit=on  SystemSampleTime=mdl.T
  x_offset : Constant  Value=rbt1.offset.x
  y_offset : Constant  Value=rbt1.offset.y
  X (m)1 : Outport
  Y (m)1 : Outport  Port=2
  Z (m)1 : Outport  Port=3
  alpha (radians)1 : Outport  Port=4
  beta (radians)1 : Outport  Port=5
  gamma (radians)1 : Outport  Port=6
  XYZ (m) : Outport  Port=7
  alphs,beta,gamma (rad) : Outport  Port=8
  enable : Outport  Port=9
  landing : Outport  Port=10
  wires:
  X(m) in/1 -> safety check system/1(x), low pass/1, envelope/voltage check/1(x), X (m)1/1
  Y(m) in/1 -> safety check system/2(y), low pass1/1, envelope/voltage check/2(y), Y (m)1/1
  Z(m) in/1 -> safety check system/3(z), low pass2/1, envelope/voltage check/3(z), Z (m)1/1
  low pass1/1 -> Mux/2
  alpha in/1 -> safety check system/4(alpha), " "/2
  beta in/1 -> "  "/1, safety check system/5(beta)
  low pass/1 -> Mux/1
  low pass2/1 -> Mux/3
  Mux/1 -> XYZ (m)/1
  Mux1/1 -> alphs,beta,gamma (rad)/1
  y_offset/1 -> "  "/2
  x_offset/1 -> " "/1
  control voltage/1 -> Delay2/1, safety check system/7(voltage)
  safety check system/1(stop_out) -> enable/1
  Gain/1 -> SaturatingRamp/1
  Data Type Conversion3/1 -> turn off memory check/1
  Data Type Conversion1/1 -> torelance time/1
  type conv/1 -> SaturatingRamp/2, Gain/1
  SaturatingRamp/1 -> Data Type Conversion1/1
  torelance time/1 -> Data Type Conversion3/1
  turn off memory check/1 -> Compare To Zero2/1, Memory/1
  Memory/1 -> turn off memory check/2
  Compare To Zero2/1 -> Data Type Conversion2/1
  " "/1 -> Mux1/1, alpha (radians)1/1
  "  "/1 -> beta (radians)1/1, Mux1/2
  gamma in/1 -> Mux1/3, gamma (radians)1/1, safety check system/6(gamma)
  Delay/1 -> MATLAB Function/3(cum_in)
  MATLAB Function/2(cum_out) -> Delay/1
  MATLAB Function/1(landing_out) -> Delay1/1, landing/1
  Delay1/1 -> MATLAB Function/2(landing_in)
  envelope/voltage check/1(keep_flying) -> Product/1
  Delay2/1 -> voltage check/1(voltage)
  voltage check/1(keep_flying) -> Product/2
  Product/1 -> MATLAB Function/1(keep_flying)

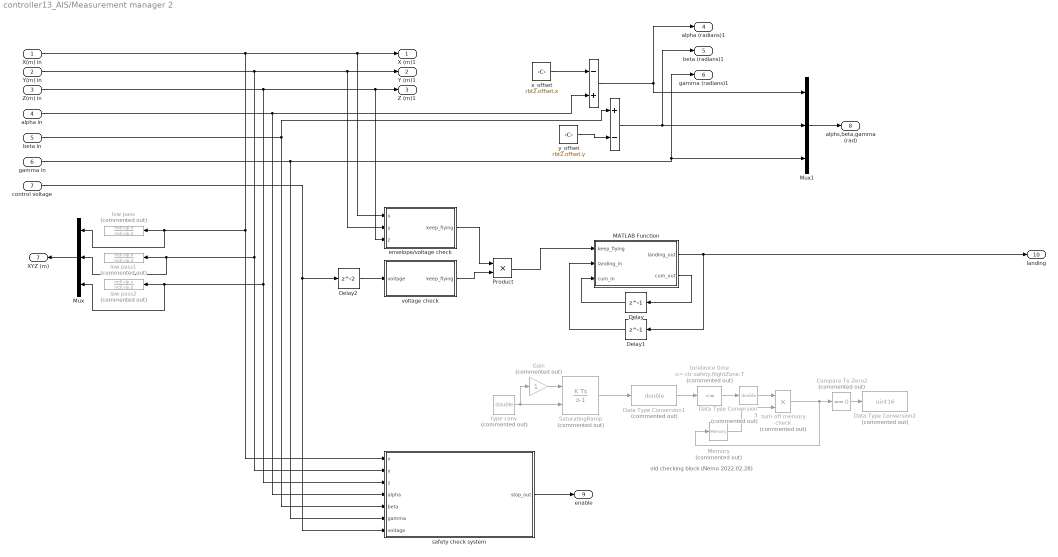
== system controller13_AIS/Measurement manager 2 ==
  note: old checking block (Nemo 2022.02.28)
  X(m) in : Inport
  Y(m) in : Inport  Port=2
  Z(m) in : Inport  Port=3
  alpha in : Inport  Port=4
  beta in : Inport  Port=5
  gamma in : Inport  Port=6
  control voltage : Inport  Port=7
  " " : Sum  Inputs=-+
  "  " : Sum  Inputs=+-
  Compare To Zero2 : simulink/Logic and Bit Operations/Compare To Zero  Commented=on  relop===  OutDataTypeStr=uint8
  Data Type Conversion1 : DataTypeConversion  Commented=on  OutDataTypeStr=double
  Data Type Conversion2 : DataTypeConversion  Commented=on  OutDataTypeStr=uint16
  Data Type Conversion3 : DataTypeConversion  Commented=on  OutDataTypeStr=double
  Delay : Delay  DelayLength=1
  Delay1 : Delay  DelayLength=1
  Delay2 : Delay
  Gain : Gain  Commented=on
  MATLAB Function : MATLAB Function  TreatAsAtomicUnit=on
  Memory : Memory  Commented=on  InitialCondition=1
  Mux : Mux  Inputs=3
  Mux1 : Mux  Inputs=3
  Product : Product
  SaturatingRamp : DiscreteIntegrator  Commented=on  gainval=1  ExternalReset=falling  SampleTime=-1  UpperSaturationLimit=1  LowerSaturationLimit=0  ICPrevOutput=DiscIntNeverNeededParam  ICPrevScaledInput=DiscIntNeverNeededParam
  envelope/voltage check : MATLAB Function  TreatAsAtomicUnit=on
  low pass : DiscreteTransferFcn  Commented=on  Numerator=mdl.vlp.n  Denominator=mdl.vlp.d
  low pass1 : DiscreteTransferFcn  Commented=on  Numerator=mdl.vlp.n  Denominator=mdl.vlp.d
  low pass2 : DiscreteTransferFcn  Commented=on  Numerator=mdl.vlp.n  Denominator=mdl.vlp.d
  safety check system : Subsystem
  torelance time : simulink/Logic and Bit Operations/Compare To Constant  Commented=on  relop=<=  const=ctr.safety.flightZone.T  OutDataTypeStr=uint8
  turn off memory check : Product  Commented=on  RndMeth=Zero
  type conv : DataTypeConversion  Commented=on  OutDataTypeStr=double
  voltage check : MATLAB Function  TreatAsAtomicUnit=on  SystemSampleTime=mdl.T
  x_offset : Constant  Value=rbt2.offset.x
  y_offset : Constant  Value=rbt2.offset.y
  X (m)1 : Outport
  Y (m)1 : Outport  Port=2
  Z (m)1 : Outport  Port=3
  alpha (radians)1 : Outport  Port=4
  beta (radians)1 : Outport  Port=5
  gamma (radians)1 : Outport  Port=6
  XYZ (m) : Outport  Port=7
  alphs,beta,gamma (rad) : Outport  Port=8
  enable : Outport  Port=9
  landing : Outport  Port=10
  wires:
  X(m) in/1 -> safety check system/1(x), Mux/1, low pass/1, envelope/voltage check/1(x), X (m)1/1
  Y(m) in/1 -> safety check system/2(y), Mux/2, low pass1/1, envelope/voltage check/2(y), Y (m)1/1
  Z(m) in/1 -> safety check system/3(z), Mux/3, low pass2/1, envelope/voltage check/3(z), Z (m)1/1
  alpha in/1 -> safety check system/4(alpha), " "/2
  beta in/1 -> "  "/1, safety check system/5(beta)
  Mux/1 -> XYZ (m)/1
  Mux1/1 -> alphs,beta,gamma (rad)/1
  y_offset/1 -> "  "/2
  x_offset/1 -> " "/1
  control voltage/1 -> Delay2/1, safety check system/7(voltage)
  safety check system/1(stop_out) -> enable/1
  Gain/1 -> SaturatingRamp/1
  Data Type Conversion3/1 -> turn off memory check/1
  Data Type Conversion1/1 -> torelance time/1
  type conv/1 -> SaturatingRamp/2, Gain/1
  SaturatingRamp/1 -> Data Type Conversion1/1
  torelance time/1 -> Data Type Conversion3/1
  turn off memory check/1 -> Compare To Zero2/1, Memory/1
  Memory/1 -> turn off memory check/2
  Compare To Zero2/1 -> Data Type Conversion2/1
  " "/1 -> Mux1/1, alpha (radians)1/1
  "  "/1 -> beta (radians)1/1, Mux1/2
  gamma in/1 -> Mux1/3, gamma (radians)1/1, safety check system/6(gamma)
  Delay/1 -> MATLAB Function/3(cum_in)
  MATLAB Function/2(cum_out) -> Delay/1
  MATLAB Function/1(landing_out) -> Delay1/1, landing/1
  Delay1/1 -> MATLAB Function/2(landing_in)
  envelope/voltage check/1(keep_flying) -> Product/1
  Delay2/1 -> voltage check/1(voltage)
  voltage check/1(keep_flying) -> Product/2
  Product/1 -> MATLAB Function/1(keep_flying)

== system controller13_AIS/Phantom trigger ==
  note: high-speed camera trigger
  Switch2 : Switch  Criteria=u2 > Threshold
  conv : DataTypeConversion  OutDataTypeStr=double
  pretrigger : Constant
  start at one : MATLAB Function  TreatAsAtomicUnit=on
  timer1 : Subsystem
  trigger_camera : Constant
  zero : Constant  Value=0
  wires:
  trigger_camera/1 -> Switch2/2
  zero/1 -> Switch2/3
  Switch2/1 -> conv/1
  start at one/1(trigger) -> Switch2/1
  timer1/1(time) -> start at one/1(time)
